simulink model "nonlineardtm"  (R2018b)
settings: configuration reference "Physics" (kept outside this file)
model workspace (MAT data in the model file):
  MCOS : class17 (value not decoded)
undefined symbols (not defined in the file): INIT__initialvalues__Vehicle_InitialPitchAngle, INIT__initialvalues__Vehicle_InitialPitchRate_radps, INIT__initialvalues__Vehicle_InitialVelocity_mps__2, INIT__initialvalues__Vehicle_InitialVelocity_mps__3, INIT__initialvalues__Vehicle_InitialYawAngle, INIT__initialvalues__Vehicle_InitialYawRate_radps, tireFL__INERTIAL__m_Wheel_kg, tireFL__SCALING__LCX, tireFL__SCALING__LCY, tireFL__SCALING__LCZ, tireFL__SCALING__LEX, tireFL__SCALING__LEY, tireFL__SCALING__LFZO, tireFL__SCALING__LGAY, tireFL__SCALING__LGAZ, tireFL__SCALING__LHX, tireFL__SCALING__LHY, tireFL__SCALING__LKX, tireFL__SCALING__LKY, tireFL__SCALING__LMPHI, tireFL__SCALING__LMUV, tireFL__SCALING__LMX, tireFL__SCALING__LMY, tireFL__SCALING__LRES, tireFL__SCALING__LS, tireFL__SCALING__LTR, tireFL__SCALING__LVMX, tireFL__SCALING__LVX, tireFL__SCALING__LVY, tireFL__SCALING__LVYKA, tireFL__SCALING__LXAL, tireFL__SCALING__LYKA, tireFR__INERTIAL__m_Wheel_kg, tireFR__SCALING__LCX, tireFR__SCALING__LCY, tireFR__SCALING__LCZ, tireFR__SCALING__LEX, tireFR__SCALING__LEY, tireFR__SCALING__LFZO, tireFR__SCALING__LGAY, tireFR__SCALING__LGAZ, tireFR__SCALING__LHX, tireFR__SCALING__LHY, tireFR__SCALING__LKX, tireFR__SCALING__LKY, tireFR__SCALING__LMPHI, tireFR__SCALING__LMUV, tireFR__SCALING__LMX, tireFR__SCALING__LMY, tireFR__SCALING__LRES, tireFR__SCALING__LS, tireFR__SCALING__LTR, tireFR__SCALING__LVMX, tireFR__SCALING__LVX, tireFR__SCALING__LVY, tireFR__SCALING__LVYKA, tireFR__SCALING__LXAL, tireFR__SCALING__LYKA, tireRL__INERTIAL__m_Wheel_kg, tireRL__SCALING__LCX ... (+71)
libraries: vehdynlibtire_TUM x4, vehdynlibsuspension x2, vrlib x1, vehdynlibeom_TUM x1
(part 3 of 5)

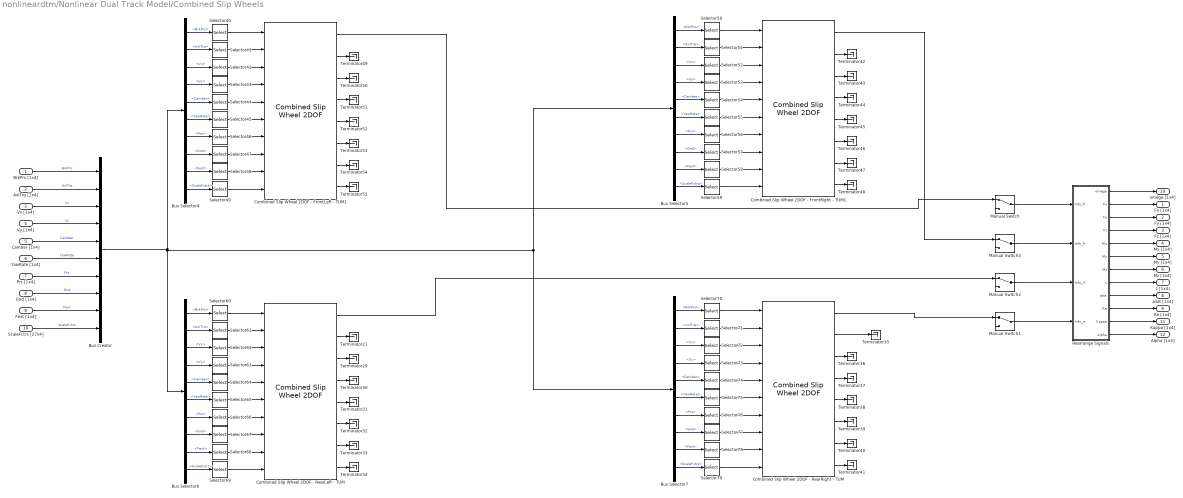
== system nonlineardtm/Nonlinear Dual Track Model/Combined Slip Wheels ==
  BrkPrs [1x4] : Inport
  AxlTrq [1x4] : Inport  Port=2
  Vx [1x4] : Inport  Port=3
  Vy [1x4] : Inport  Port=4
  Camber [1x4] : Inport  Port=5
  YawRate [1x4] : Inport  Port=6
  Prs [1x4] : Inport  Port=7
  Gnd [1x4] : Inport  Port=8
  Fext [1x4] : Inport  Port=9
  ScaleFctrs [27x4] : Inport  Port=10
  Bus Creator : BusCreator  Inputs=10
  Bus Selector{4..7} (4 alike) : BusSelector  OutputSignals=BrkPrs,AxlTrq,Vx,Vy,Camber,YawRate,Prs,Gnd,Fext,ScaleFctrs
  Combined Slip Wheel 2DOF - FrontLeft - TUM1 : vehdynlibtire_TUM/Combined Slip Wheel 2DOF  BrakeType=Disc  mu_static=VEH__Brakes__mue_BrakePadsFrRe_static__1  mu_kinetic=VEH__Brakes__mue_BrakePadsFrRe_kinetic__1  disk_abore=VEH__Brakes__d_BrakeActuatorBoreFrRe_m__1  Rm=VEH__Brakes__r_BrakePadsMeanLeverFrRe_m__1  num_pads=VEH__Brakes__n_BrakePadsNumberFrRe__1  drum_abore=0.0508  drum_a=0.123  drum_c=0.212  drum_r=0.15  drum_theta1=0  drum_theta2=126  brake_p_bpt=[1 11.4736842105263 21.9473684210526 32.4210526315789 42.8947368421053 53.3684210526316 63.8421052631579 74.3157894736842 84.7894736842105 95.2631578947368 105.736842105263 116.210526315789 126.684210526316 137.157894736842 147.631578947368 158.105263157895 168.578947368421 179.052631578947 189.526315789474 200]  brake_n_bpt=[0 52.6315789473684 105.263157894737 157.894736842105 210.526315789474 263.157894736842 315.789473684211 368.421052631579 421.052631578947 473.684210526316 526.315789473684 578.947368421053 631.578947368421 684.210526315789 736.842105263158 789.473684210526 842.105263157895 894.736842105263 947.368421052632 1000]  f_brake_t=[43.4900602404453 42.5056030554862 41.5350898940194 40.5780454442085 39.6340111501808 38.7025443887544 37.7832176914519 36.8756180088306 35.9793460143796 35.0940154454303 34.2192524787115 33.3546951383474 32.4999927342521 31.6548053290159 30.8188032315107 29.991666515561 29.1730845621415 28.362755623661 27.5603864089927 26.765691687993;498.991217495636 487.695866636631 476.560505099801 465.579679307235 454.748127933653 444.060772460445 433.51270824929 423.099196101319 412.81565427025 402.657650900201 392.620896861006 382.701238955775 372.894653477208 363.197240090814 353.605216024701 344.114910546964 334.722759712992 325.425301366216 316.219170376863 307.10109410434;954.492374750826 932.886130217776 911.585920305583 890.581313170261 869.862244717126 849.419000532136 829.242198807128 809.322774193808 789.651962526121 770.221286354971 751.0225412433 732.047782773203 713.289314220164 694.739674852612 676.391628817892 658.238154578366 640.272434863842 622.48784710877 604.877954344734 587.436496520688;1409.99353200602 1378.07639379892 1346.61133551136 1315.58294703329 1284.9763615006 1254.77722860383 1224.97168936497 1195.5463522863 1166.48827078199 1137.78492180974 1109.42418562559 1081.39432659063 1053.68397496312 1026.28210961441 999.178041611083 972.361398609768 945.822110014692 919.550392851325 893.536738312604 867.771898937035;1865.49468926121 1823.26665738007 1781.63675071715 1740.58458089631 1700.09047828407 1660.13545667552 1620.7011799228 1581.76993037878 1543.32457903786 1505.34855726451 1467.82583000789 1430.74087040806 1394.07863570608 1357.82454437621 1321.96445440427 1286.48464264117 1251.37178516554 1216.61293859388 1182.19552228048 1148.10730135338;2320.9958465164 2268.45692096121 2216.66216592293 2165.58621475934 2115.20459506754 2065.49368474721 2016.43067048064 1967.99350847127 1920.16088729373 1872.91219271928 1826.22747439018 1780.08741422549 1734.47329644903 1689.36697913801 1644.75086719747 1600.60788667257 1556.92146031639 1513.67548433643 1470.85430624835 1428.44270376973;2776.49700377159 2713.64718454235 2651.68758112871 2590.58784862237 2530.31871185102 2470.8519128189 2412.16016103848 2354.21708656376 2296.9971955496 2240.47582817405 2184.62911877248 2129.43395804292 2074.86795719199 2020.9094138998 1967.53727999066 1914.73113070398 1862.47113546724 1810.73803007899 1759.51309021622 1708.77810618608;3231.99816102678 3158.8374481235 3086.71299633449 3015.58948248539 2945.43282863449 2876.21014089059 2807.88965159632 2740.44066465625 2673.83350380547 2608.03946362882 2543.03076315477 2478.78050186034 2415.26261793494 2352.4518486616 2290.32369278385 2228.85437473538 2168.02081061809 2107.80057582154 2048.17187418409 1989.11350860242;3687.49931828197 3604.02771170464 3521.73841154027 3440.59111634842 3360.54694541796 3281.56836896228 3203.61914215416 3126.66424274874 3050.66981206134 2975.60309908359 2901.43240753707 2828.12704567777 2755.6572786779 2683.9942834234 2613.11010557704 2542.97761876678 2473.57048576894 2404.8631215641 2336.83065815196 2269.44891101877;4143.00047553716 4049.21797528579 3956.76382674606 3865.59275021144 3775.66106220143 3686.92659703397 3599.34863271199 3512.88782084123 3427.50612031721 3343.16673453836 3259.83405191936 3177.4735894952 3096.05193942085 3015.5367181852 2935.89651837023 2857.10086279818 2779.12016091979 2701.92566730665 2625.48944211983 2549.78431343512;4598.50163279235 4494.40823886693 4391.78924195184 4290.59438407447 4190.77517898491 4092.28482510566 3995.07812326983 3899.11139893372 3804.34242857308 3710.73036999313 3618.23569630166 3526.82013331263 3436.44660016381 3347.079152947 3258.68293116342 3171.22410682959 3084.66983607064 2998.98821304921 2914.1482260877 2830.11971585147;5054.00279004754 4939.59850244808 4826.81465715762 4715.59601793749 4605.88929576838 4497.64305317735 4390.80761382767 4285.3349770262 4181.17873682896 4078.2940054479 3976.63734068395 3876.16667713006 3776.84126090677 3678.62158770879 3581.46934395661 3485.34735086099 ...(+2764 chars)]  tireParamSet=vdynPassCar.mat  plySteer=off  turnslip=off  PRESMAX=tireFL__SIMULATION__PRESMAX  PRESMIN=tireFL__SIMULATION__PRESMIN  FZMAX=tireFL__SIMULATION__FZMAX  FZMIN=tireFL__SIMULATION__FZMIN  VXLOW=tireFL__SIMULATION__VXLOW  KPUMAX=tireFL__SIMULATION__KPUMAX  KPUMIN=tireFL__SIMULATION__KPUMIN  ALPMAX=tireFL__SIMULATION__ALPMAX  ALPMIN=tireFL__SIMULATION__ALPMIN  CAMMAX=tireFL__SIMULATION__CAMMAX  CAMMIN=tireFL__SIMULATION__CAMMIN  LONGVL=tireFL__SIMULATION__LONGVL  omegao=INIT__initialvalues__omega0_Wheels_radps__1  br=tireFL__WHEEL__br_Nmsprad  UNLOADED_RADIUS=tireFL__WHEEL__TYRE_RADIUS_MOD  NOMPRES=tireFL__WHEEL__NORMPRES  FNOMIN=tireFL__WHEEL__FNOMIN  WIDTH=tireFL__DIMENSION__WIDTH  T_RelaxationLong=tireFL__WHEEL__T_RelaxationLong  T_RelaxationLat=tireFL__WHEEL__T_RelaxationLat  T_RelaxationMy=tireFL__WHEEL__T_RelaxationMy  MASS=tireFL__INERTIAL__m_Wheel_kg  IYY=tireFL__INERTIAL__Iyy_Wheel_kgm2  GRAVITY=- VEH__Environment__a_Gravity_mps2  zo=INIT__initialvalues__z0_TireDeflection_m__1  zdoto=INIT__initialvalues__v0z_Wheels_mps__1  BREFF=tireFL__VERTICAL__BREFF  DREFF=tireFL__VERTICAL__DREFF  FREFF=tireFL__VERTICAL__FREFF  Q_RE0=tireFL__VERTICAL__Q_RE0  Q_V1=tireFL__VERTICAL__Q_V1  Q_V2=tireFL__VERTICAL__Q_V2  Q_FZ1=tireFL__VERTICAL__Q_FZ1  Q_FZ2=tireFL__VERTICAL__Q_FZ2  Q_FZ3=tireFL__VERTICAL__Q_FZ3  Q_FCX=tireFL__VERTICAL__Q_FCX  Q_FCY=tireFL__VERTICAL__Q_FCY  Q_FCY2=tireFL__VERTICAL__Q_FCY2  PFZ1=tireFL__VERTICAL__PFZ1  VERTICAL_STIFFNESS=tireFL__VERTICAL__VERTICAL_STIFFNESS  VERTICAL_DAMPING=tireFL__VERTICAL__VERTICAL_DAMPING  LONGITUDINAL_STIFFNESS=tireFL__STRUCTURAL__LONGITUDINAL_STIFFNESS  LATERAL_STIFFNESS=tireFL__STRUCTURAL__LATERAL_STIFFNESS  PCFX1=tireFL__STRUCTURAL__PCFX1  PCFX2=tireFL__STRUCTURAL__PCFX2  PCFX3=tireFL__STRUCTURAL__PCFX3  PCFY1=tireFL__STRUCTURAL__PCFY1  PCFY2=tireFL__STRUCTURAL__PCFY2  PCFY3=tireFL__STRUCTURAL__PCFY3  Q_RA1=tireFL__CONTACTPATCH__Q_RA1  Q_RA2=tireFL__CONTACTPATCH__Q_RA2  Q_RB1=tireFL__CONTACTPATCH__Q_RB1  Q_RB2=tireFL__CONTACTPATCH__Q_RB2  PCX1=tireFL__LONGITUDINAL__PCX1  PDX1=tireFL__LONGITUDINAL__PDX1  PDX2=tireFL__LONGITUDINAL__PDX2  PDX3=tireFL__LONGITUDINAL__PDX3  PEX1=tireFL__LONGITUDINAL__PEX1  PEX2=tireFL__LONGITUDINAL__PEX2  PEX3=tireFL__LONGITUDINAL__PEX3  PEX4=tireFL__LONGITUDINAL__PEX4  PKX1=tireFL__LONGITUDINAL__PKX1  PKX2=tireFL__LONGITUDINAL__PKX2  PKX3=tireFL__LONGITUDINAL__PKX3  PHX1=tireFL__LONGITUDINAL__PHX1  PHX2=tireFL__LONGITUDINAL__PHX2  PVX1=tireFL__LONGITUDINAL__PVX1  PVX2=tireFL__LONGITUDINAL__PVX2  PPX1=tireFL__LONGITUDINAL__PPX1  PPX2=tireFL__LONGITUDINAL__PPX2  PPX3=tireFL__LONGITUDINAL__PPX3  PPX4=tireFL__LONGITUDINAL__PPX4  RBX1=tireFL__LONGITUDINAL__RBX1  RBX2=tireFL__LONGITUDINAL__RBX2  RBX3=tireFL__LONGITUDINAL__RBX3  RCX1=tireFL__LONGITUDINAL__RCX1  REX1=tireFL__LONGITUDINAL__REX1  REX2=tireFL__LONGITUDINAL__REX2  RHX1=tireFL__LONGITUDINAL__RHX1  QSX1=tireFL__OVERTURNING__QSX1  QSX2=tireFL__OVERTURNING__QSX2  QSX3=tireFL__OVERTURNING__QSX3  QSX4=tireFL__OVERTURNING__QSX4  QSX5=tireFL__OVERTURNING__QSX5  QSX6=tireFL__OVERTURNING__QSX6  QSX7=tireFL__OVERTURNING__QSX7  QSX8=tireFL__OVERTURNING__QSX8  QSX9=tireFL__OVERTURNING__QSX9  QSX10=tireFL__OVERTURNING__QSX10  QSX11=tireFL__OVERTURNING__QSX11  QSX12=tireFL__OVERTURNING__QSX12  QSX13=tireFL__OVERTURNING__QSX13  QSX14=tireFL__OVERTURNING__QSX14  PPMX1=tireFL__OVERTURNING__PPMX1  PCY1=tireFL__LATERAL__PCY1  PDY1=tireFL__LATERAL__PDY1  PDY2=tireFL__LATERAL__PDY2  PDY3=tireFL__LATERAL__PDY3  PEY1=tireFL__LATERAL__PEY1  PEY2=tireFL__LATERAL__PEY2  PEY3=tireFL__LATERAL__PEY3  PEY4=tireFL__LATERAL__PEY4  PEY5=tireFL__LATERAL__PEY5  PKY1=tireFL__LATERAL__PKY1  PKY2=tireFL__LATERAL__PKY2  PKY3=tireFL__LATERAL__PKY3  PKY4=tireFL__LATERAL__PKY4  PKY5=tireFL__LATERAL__PKY5  PKY6=tireFL__LATERAL__PKY6  PKY7=tireFL__LATERAL__PKY7  PHY1=tireFL__LATERAL__PHY1  PHY2=tireFL__LATERAL__PHY2  PVY1=tireFL__LATERAL__PVY1  PVY2=tireFL__LATERAL__PVY2  PVY3=tireFL__LATERAL__PVY3  PVY4=tireFL__LATERAL__PVY4  PPY1=tireFL__LATERAL__PPY1  PPY2=tireFL__LATERAL__PPY2  PPY3=tireFL__LATERAL__PPY3  PPY4=tireFL__LATERAL__PPY4  PPY5=tireFL__LATERAL__PPY5  RBY1=tireFL__LATERAL__RBY1  RBY2=tireFL__LATERAL__RBY2  RBY3=tireFL__LATERAL__RBY3  RBY4=tireFL__LATERAL__RBY4  RCY1=tireFL__LATERAL__RCY1  REY1=tireFL__LATERAL__REY1  REY2=tireFL__LATERAL__REY2  RHY1=tireFL__LATERAL__RHY1  RHY2=tireFL__LATERAL__RHY2  RVY1=tireFL__LATERAL__RVY1  RVY2=tireFL__LATERAL__RVY2  RVY3=tireFL__LATERAL__RVY3  RVY4=tireFL__LATERAL__RVY4  RVY5=tireFL__LATERAL__RVY5  RVY6=tireFL__LATERAL__RVY6  QSY1=tireFL__ROLLING__QSY1  QSY2=tireFL__ROLLING__QSY2  QSY3=tireFL__ROLLING__QSY3  QSY4=tireFL__ROLLING__QSY4  QSY5=tireFL__ROLLING__QSY5  QSY6=tireFL__ROLLING__QSY6  QSY7=tireFL__ROLLING__QSY7  QSY8=tireFL__ROLLING__QSY8  QBZ1=tireFL__ALIGNING__QBZ1  QBZ2=tireFL__ALIGNING__QBZ2  QBZ3=tireFL__ALIGNING__QBZ3  QBZ4=tireFL__ALIGNING__QBZ4  QBZ5=tireFL__ALIGNING__QBZ5  QBZ6=tireFL__ALIGNING__QBZ6  QBZ9=tireFL__ALIGNING__QBZ9  QBZ10=tireFL__ALIGNING__QBZ10  QCZ1=tireFL__ALIGNING__QCZ1  QDZ1=tireFL__ALIGNING__QDZ1  QDZ2=tireFL__ALIGNING__QDZ2  QDZ3=tireFL__ALIGNING__QDZ3  QDZ4=tireFL__ALIGNING__QDZ4  QDZ6=tireFL__ALIGNING__QDZ6  QDZ7=tireFL__ALIGNING__QDZ7  QDZ8=tireFL__ALIGNING__QDZ8  QDZ9=tireFL__ALIGNING__QDZ9  QDZ10=tireFL__ALIGNING__QDZ10  QDZ11=tireFL__ALIGNING__QDZ11  QEZ1=tireFL__ALIGNING__QEZ1  QEZ2=tireFL__ALIGNING__QEZ2  QEZ3=tireFL__ALIGNING__QEZ3  QEZ4=tireFL__ALIGNING__QEZ4  QEZ5=tireFL__ALIGNING__QEZ5  QHZ1=tireFL__ALIGNING__QHZ1  QHZ2=tireFL__ALIGNING__QHZ2  QHZ3=tireFL__ALIGNING__QHZ3  QHZ4=tireFL__ALIGNING__QHZ4  PPZ1=tireFL__ALIGNING__PPZ1  PPZ2=tireFL__ALIGNING__PPZ2  SSZ1=tireFL__ALIGNING__SSZ1  SSZ2=tireFL__ALIGNING__SSZ2  SSZ3=tireFL__ALIGNING__SSZ3  SSZ4=tireFL__ALIGNING__SSZ4  PDXP1=tireFL__TURNSLIP__PDXP1  PDXP2=tireFL__TURNSLIP__PDXP2  PDXP3=tireFL__TURNSLIP__PDXP3  PKYP1=tireFL__TURNSLIP__PKYP1  PDYP1=tireFL__TURNSLIP__PDYP1  PDYP2=tireFL__TURNSLIP__PDYP2  PDYP3=tireFL__TURNSLIP__PDYP3  PDYP4=tireFL__TURNSLIP__PDYP4  PHYP1=tireFL__TURNSLIP__PHYP1  PHYP2=tireFL__TURNSLIP__PHYP2  PHYP3=tireFL__TURNSLIP__PHYP3  PHYP4=tireFL__TURNSLIP__PHYP4  PECP1=tireFL__TURNSLIP__PECP1  PECP2=tireFL__TURNSLIP__PECP2  QDTP1=tireFL__TURNSLIP__QDTP1  QCRP1=tireFL__TURNSLIP__QCRP1  QCRP2=tireFL__TURNSLIP__QCRP2  QBRP1=tireFL__TURNSLIP__QBRP1  QDRP1=tireFL__TURNSLIP__QDRP1  QDRP2=tireFL__TURNSLIP__QDRP2  aMode=2
  Combined Slip Wheel 2DOF - FrontRight - TUM1 : vehdynlibtire_TUM/Combined Slip Wheel 2DOF  BrakeType=Disc  mu_static=VEH__Brakes__mue_BrakePadsFrRe_static__1  mu_kinetic=VEH__Brakes__mue_BrakePadsFrRe_kinetic__1  disk_abore=VEH__Brakes__d_BrakeActuatorBoreFrRe_m__1  Rm=VEH__Brakes__r_BrakePadsMeanLeverFrRe_m__1  num_pads=VEH__Brakes__n_BrakePadsNumberFrRe__1  drum_abore=0.0508  drum_a=0.123  drum_c=0.212  drum_r=0.15  drum_theta1=0  drum_theta2=126  brake_p_bpt=[1 11.4736842105263 21.9473684210526 32.4210526315789 42.8947368421053 53.3684210526316 63.8421052631579 74.3157894736842 84.7894736842105 95.2631578947368 105.736842105263 116.210526315789 126.684210526316 137.157894736842 147.631578947368 158.105263157895 168.578947368421 179.052631578947 189.526315789474 200]  brake_n_bpt=[0 52.6315789473684 105.263157894737 157.894736842105 210.526315789474 263.157894736842 315.789473684211 368.421052631579 421.052631578947 473.684210526316 526.315789473684 578.947368421053 631.578947368421 684.210526315789 736.842105263158 789.473684210526 842.105263157895 894.736842105263 947.368421052632 1000]  f_brake_t=[43.4900602404453 42.5056030554862 41.5350898940194 40.5780454442085 39.6340111501808 38.7025443887544 37.7832176914519 36.8756180088306 35.9793460143796 35.0940154454303 34.2192524787115 33.3546951383474 32.4999927342521 31.6548053290159 30.8188032315107 29.991666515561 29.1730845621415 28.362755623661 27.5603864089927 26.765691687993;498.991217495636 487.695866636631 476.560505099801 465.579679307235 454.748127933653 444.060772460445 433.51270824929 423.099196101319 412.81565427025 402.657650900201 392.620896861006 382.701238955775 372.894653477208 363.197240090814 353.605216024701 344.114910546964 334.722759712992 325.425301366216 316.219170376863 307.10109410434;954.492374750826 932.886130217776 911.585920305583 890.581313170261 869.862244717126 849.419000532136 829.242198807128 809.322774193808 789.651962526121 770.221286354971 751.0225412433 732.047782773203 713.289314220164 694.739674852612 676.391628817892 658.238154578366 640.272434863842 622.48784710877 604.877954344734 587.436496520688;1409.99353200602 1378.07639379892 1346.61133551136 1315.58294703329 1284.9763615006 1254.77722860383 1224.97168936497 1195.5463522863 1166.48827078199 1137.78492180974 1109.42418562559 1081.39432659063 1053.68397496312 1026.28210961441 999.178041611083 972.361398609768 945.822110014692 919.550392851325 893.536738312604 867.771898937035;1865.49468926121 1823.26665738007 1781.63675071715 1740.58458089631 1700.09047828407 1660.13545667552 1620.7011799228 1581.76993037878 1543.32457903786 1505.34855726451 1467.82583000789 1430.74087040806 1394.07863570608 1357.82454437621 1321.96445440427 1286.48464264117 1251.37178516554 1216.61293859388 1182.19552228048 1148.10730135338;2320.9958465164 2268.45692096121 2216.66216592293 2165.58621475934 2115.20459506754 2065.49368474721 2016.43067048064 1967.99350847127 1920.16088729373 1872.91219271928 1826.22747439018 1780.08741422549 1734.47329644903 1689.36697913801 1644.75086719747 1600.60788667257 1556.92146031639 1513.67548433643 1470.85430624835 1428.44270376973;2776.49700377159 2713.64718454235 2651.68758112871 2590.58784862237 2530.31871185102 2470.8519128189 2412.16016103848 2354.21708656376 2296.9971955496 2240.47582817405 2184.62911877248 2129.43395804292 2074.86795719199 2020.9094138998 1967.53727999066 1914.73113070398 1862.47113546724 1810.73803007899 1759.51309021622 1708.77810618608;3231.99816102678 3158.8374481235 3086.71299633449 3015.58948248539 2945.43282863449 2876.21014089059 2807.88965159632 2740.44066465625 2673.83350380547 2608.03946362882 2543.03076315477 2478.78050186034 2415.26261793494 2352.4518486616 2290.32369278385 2228.85437473538 2168.02081061809 2107.80057582154 2048.17187418409 1989.11350860242;3687.49931828197 3604.02771170464 3521.73841154027 3440.59111634842 3360.54694541796 3281.56836896228 3203.61914215416 3126.66424274874 3050.66981206134 2975.60309908359 2901.43240753707 2828.12704567777 2755.6572786779 2683.9942834234 2613.11010557704 2542.97761876678 2473.57048576894 2404.8631215641 2336.83065815196 2269.44891101877;4143.00047553716 4049.21797528579 3956.76382674606 3865.59275021144 3775.66106220143 3686.92659703397 3599.34863271199 3512.88782084123 3427.50612031721 3343.16673453836 3259.83405191936 3177.4735894952 3096.05193942085 3015.5367181852 2935.89651837023 2857.10086279818 2779.12016091979 2701.92566730665 2625.48944211983 2549.78431343512;4598.50163279235 4494.40823886693 4391.78924195184 4290.59438407447 4190.77517898491 4092.28482510566 3995.07812326983 3899.11139893372 3804.34242857308 3710.73036999313 3618.23569630166 3526.82013331263 3436.44660016381 3347.079152947 3258.68293116342 3171.22410682959 3084.66983607064 2998.98821304921 2914.1482260877 2830.11971585147;5054.00279004754 4939.59850244808 4826.81465715762 4715.59601793749 4605.88929576838 4497.64305317735 4390.80761382767 4285.3349770262 4181.17873682896 4078.2940054479 3976.63734068395 3876.16667713006 3776.84126090677 3678.62158770879 3581.46934395661 3485.34735086099 ...(+2764 chars)]  tireParamSet=vdynPassCar.mat  plySteer=off  turnslip=off  PRESMAX=tireFR__SIMULATION__PRESMAX  PRESMIN=tireFR__SIMULATION__PRESMIN  FZMAX=tireFR__SIMULATION__FZMAX  FZMIN=tireFR__SIMULATION__FZMIN  VXLOW=tireFR__SIMULATION__VXLOW  KPUMAX=tireFR__SIMULATION__KPUMAX  KPUMIN=tireFR__SIMULATION__KPUMIN  ALPMAX=tireFR__SIMULATION__ALPMAX  ALPMIN=tireFR__SIMULATION__ALPMIN  CAMMAX=tireFR__SIMULATION__CAMMAX  CAMMIN=tireFR__SIMULATION__CAMMIN  LONGVL=tireFR__SIMULATION__LONGVL  omegao=INIT__initialvalues__omega0_Wheels_radps__2  br=tireFR__WHEEL__br_Nmsprad  UNLOADED_RADIUS=tireFR__WHEEL__TYRE_RADIUS_MOD  NOMPRES=tireFR__WHEEL__NORMPRES  FNOMIN=tireFR__WHEEL__FNOMIN  WIDTH=tireFR__DIMENSION__WIDTH  T_RelaxationLong=tireFR__WHEEL__T_RelaxationLong  T_RelaxationLat=tireFR__WHEEL__T_RelaxationLat  T_RelaxationMy=tireFR__WHEEL__T_RelaxationMy  MASS=tireFR__INERTIAL__m_Wheel_kg  IYY=tireFR__INERTIAL__Iyy_Wheel_kgm2  GRAVITY=- VEH__Environment__a_Gravity_mps2  zo=INIT__initialvalues__z0_TireDeflection_m__2  zdoto=INIT__initialvalues__v0z_Wheels_mps__2  BREFF=tireFR__VERTICAL__BREFF  DREFF=tireFR__VERTICAL__DREFF  FREFF=tireFR__VERTICAL__FREFF  Q_RE0=tireFR__VERTICAL__Q_RE0  Q_V1=tireFR__VERTICAL__Q_V1  Q_V2=tireFR__VERTICAL__Q_V2  Q_FZ1=tireFR__VERTICAL__Q_FZ1  Q_FZ2=tireFR__VERTICAL__Q_FZ2  Q_FZ3=tireFR__VERTICAL__Q_FZ3  Q_FCX=tireFR__VERTICAL__Q_FCX  Q_FCY=tireFR__VERTICAL__Q_FCY  Q_FCY2=tireFR__VERTICAL__Q_FCY2  PFZ1=tireFR__VERTICAL__PFZ1  VERTICAL_STIFFNESS=tireFR__VERTICAL__VERTICAL_STIFFNESS  VERTICAL_DAMPING=tireFR__VERTICAL__VERTICAL_DAMPING  LONGITUDINAL_STIFFNESS=tireFR__STRUCTURAL__LONGITUDINAL_STIFFNESS  LATERAL_STIFFNESS=tireFR__STRUCTURAL__LATERAL_STIFFNESS  PCFX1=tireFR__STRUCTURAL__PCFX1  PCFX2=tireFR__STRUCTURAL__PCFX2  PCFX3=tireFR__STRUCTURAL__PCFX3  PCFY1=tireFR__STRUCTURAL__PCFY1  PCFY2=tireFR__STRUCTURAL__PCFY2  PCFY3=tireFR__STRUCTURAL__PCFY3  Q_RA1=tireFR__CONTACTPATCH__Q_RA1  Q_RA2=tireFR__CONTACTPATCH__Q_RA2  Q_RB1=tireFR__CONTACTPATCH__Q_RB1  Q_RB2=tireFR__CONTACTPATCH__Q_RB2  PCX1=tireFR__LONGITUDINAL__PCX1  PDX1=tireFR__LONGITUDINAL__PDX1  PDX2=tireFR__LONGITUDINAL__PDX2  PDX3=tireFR__LONGITUDINAL__PDX3  PEX1=tireFR__LONGITUDINAL__PEX1  PEX2=tireFR__LONGITUDINAL__PEX2  PEX3=tireFR__LONGITUDINAL__PEX3  PEX4=tireFR__LONGITUDINAL__PEX4  PKX1=tireFR__LONGITUDINAL__PKX1  PKX2=tireFR__LONGITUDINAL__PKX2  PKX3=tireFR__LONGITUDINAL__PKX3  PHX1=tireFR__LONGITUDINAL__PHX1  PHX2=tireFR__LONGITUDINAL__PHX2  PVX1=tireFR__LONGITUDINAL__PVX1  PVX2=tireFR__LONGITUDINAL__PVX2  PPX1=tireFR__LONGITUDINAL__PPX1  PPX2=tireFR__LONGITUDINAL__PPX2  PPX3=tireFR__LONGITUDINAL__PPX3  PPX4=tireFR__LONGITUDINAL__PPX4  RBX1=tireFR__LONGITUDINAL__RBX1  RBX2=tireFR__LONGITUDINAL__RBX2  RBX3=tireFR__LONGITUDINAL__RBX3  RCX1=tireFR__LONGITUDINAL__RCX1  REX1=tireFR__LONGITUDINAL__REX1  REX2=tireFR__LONGITUDINAL__REX2  RHX1=tireFR__LONGITUDINAL__RHX1  QSX1=tireFR__OVERTURNING__QSX1  QSX2=tireFR__OVERTURNING__QSX2  QSX3=tireFR__OVERTURNING__QSX3  QSX4=tireFR__OVERTURNING__QSX4  QSX5=tireFR__OVERTURNING__QSX5  QSX6=tireFR__OVERTURNING__QSX6  QSX7=tireFR__OVERTURNING__QSX7  QSX8=tireFR__OVERTURNING__QSX8  QSX9=tireFR__OVERTURNING__QSX9  QSX10=tireFR__OVERTURNING__QSX10  QSX11=tireFR__OVERTURNING__QSX11  QSX12=tireFR__OVERTURNING__QSX12  QSX13=tireFR__OVERTURNING__QSX13  QSX14=tireFR__OVERTURNING__QSX14  PPMX1=tireFR__OVERTURNING__PPMX1  PCY1=tireFR__LATERAL__PCY1  PDY1=tireFR__LATERAL__PDY1  PDY2=tireFR__LATERAL__PDY2  PDY3=tireFR__LATERAL__PDY3  PEY1=tireFR__LATERAL__PEY1  PEY2=tireFR__LATERAL__PEY2  PEY3=tireFR__LATERAL__PEY3  PEY4=tireFR__LATERAL__PEY4  PEY5=tireFR__LATERAL__PEY5  PKY1=tireFR__LATERAL__PKY1  PKY2=tireFR__LATERAL__PKY2  PKY3=tireFR__LATERAL__PKY3  PKY4=tireFR__LATERAL__PKY4  PKY5=tireFR__LATERAL__PKY5  PKY6=tireFR__LATERAL__PKY6  PKY7=tireFR__LATERAL__PKY7  PHY1=tireFR__LATERAL__PHY1  PHY2=tireFR__LATERAL__PHY2  PVY1=tireFR__LATERAL__PVY1  PVY2=tireFR__LATERAL__PVY2  PVY3=tireFR__LATERAL__PVY3  PVY4=tireFR__LATERAL__PVY4  PPY1=tireFR__LATERAL__PPY1  PPY2=tireFR__LATERAL__PPY2  PPY3=tireFR__LATERAL__PPY3  PPY4=tireFR__LATERAL__PPY4  PPY5=tireFR__LATERAL__PPY5  RBY1=tireFR__LATERAL__RBY1  RBY2=tireFR__LATERAL__RBY2  RBY3=tireFR__LATERAL__RBY3  RBY4=tireFR__LATERAL__RBY4  RCY1=tireFR__LATERAL__RCY1  REY1=tireFR__LATERAL__REY1  REY2=tireFR__LATERAL__REY2  RHY1=tireFR__LATERAL__RHY1  RHY2=tireFR__LATERAL__RHY2  RVY1=tireFR__LATERAL__RVY1  RVY2=tireFR__LATERAL__RVY2  RVY3=tireFR__LATERAL__RVY3  RVY4=tireFR__LATERAL__RVY4  RVY5=tireFR__LATERAL__RVY5  RVY6=tireFR__LATERAL__RVY6  QSY1=tireFR__ROLLING__QSY1  QSY2=tireFR__ROLLING__QSY2  QSY3=tireFR__ROLLING__QSY3  QSY4=tireFR__ROLLING__QSY4  QSY5=tireFR__ROLLING__QSY5  QSY6=tireFR__ROLLING__QSY6  QSY7=tireFR__ROLLING__QSY7  QSY8=tireFR__ROLLING__QSY8  QBZ1=tireFR__ALIGNING__QBZ1  QBZ2=tireFR__ALIGNING__QBZ2  QBZ3=tireFR__ALIGNING__QBZ3  QBZ4=tireFR__ALIGNING__QBZ4  QBZ5=tireFR__ALIGNING__QBZ5  QBZ6=tireFR__ALIGNING__QBZ6  QBZ9=tireFR__ALIGNING__QBZ9  QBZ10=tireFR__ALIGNING__QBZ10  QCZ1=tireFR__ALIGNING__QCZ1  QDZ1=tireFR__ALIGNING__QDZ1  QDZ2=tireFR__ALIGNING__QDZ2  QDZ3=tireFR__ALIGNING__QDZ3  QDZ4=tireFR__ALIGNING__QDZ4  QDZ6=tireFR__ALIGNING__QDZ6  QDZ7=tireFR__ALIGNING__QDZ7  QDZ8=tireFR__ALIGNING__QDZ8  QDZ9=tireFR__ALIGNING__QDZ9  QDZ10=tireFR__ALIGNING__QDZ10  QDZ11=tireFR__ALIGNING__QDZ11  QEZ1=tireFR__ALIGNING__QEZ1  QEZ2=tireFR__ALIGNING__QEZ2  QEZ3=tireFR__ALIGNING__QEZ3  QEZ4=tireFR__ALIGNING__QEZ4  QEZ5=tireFR__ALIGNING__QEZ5  QHZ1=tireFR__ALIGNING__QHZ1  QHZ2=tireFR__ALIGNING__QHZ2  QHZ3=tireFR__ALIGNING__QHZ3  QHZ4=tireFR__ALIGNING__QHZ4  PPZ1=tireFR__ALIGNING__PPZ1  PPZ2=tireFR__ALIGNING__PPZ2  SSZ1=tireFR__ALIGNING__SSZ1  SSZ2=tireFR__ALIGNING__SSZ2  SSZ3=tireFR__ALIGNING__SSZ3  SSZ4=tireFR__ALIGNING__SSZ4  PDXP1=tireFR__TURNSLIP__PDXP1  PDXP2=tireFR__TURNSLIP__PDXP2  PDXP3=tireFR__TURNSLIP__PDXP3  PKYP1=tireFR__TURNSLIP__PKYP1  PDYP1=tireFR__TURNSLIP__PDYP1  PDYP2=tireFR__TURNSLIP__PDYP2  PDYP3=tireFR__TURNSLIP__PDYP3  PDYP4=tireFR__TURNSLIP__PDYP4  PHYP1=tireFR__TURNSLIP__PHYP1  PHYP2=tireFR__TURNSLIP__PHYP2  PHYP3=tireFR__TURNSLIP__PHYP3  PHYP4=tireFR__TURNSLIP__PHYP4  PECP1=tireFR__TURNSLIP__PECP1  PECP2=tireFR__TURNSLIP__PECP2  QDTP1=tireFR__TURNSLIP__QDTP1  QCRP1=tireFR__TURNSLIP__QCRP1  QCRP2=tireFR__TURNSLIP__QCRP2  QBRP1=tireFR__TURNSLIP__QBRP1  QDRP1=tireFR__TURNSLIP__QDRP1  QDRP2=tireFR__TURNSLIP__QDRP2  aMode=2
  Combined Slip Wheel 2DOF - RearLeft - TUM : vehdynlibtire_TUM/Combined Slip Wheel 2DOF  BrakeType=Disc  mu_static=VEH__Brakes__mue_BrakePadsFrRe_static__2  mu_kinetic=VEH__Brakes__mue_BrakePadsFrRe_kinetic__2  disk_abore=VEH__Brakes__d_BrakeActuatorBoreFrRe_m__2  Rm=VEH__Brakes__r_BrakePadsMeanLeverFrRe_m__2  num_pads=VEH__Brakes__n_BrakePadsNumberFrRe__2  drum_abore=0.0508  drum_a=0.123  drum_c=0.212  drum_r=0.15  drum_theta1=0  drum_theta2=126  brake_p_bpt=[1 11.4736842105263 21.9473684210526 32.4210526315789 42.8947368421053 53.3684210526316 63.8421052631579 74.3157894736842 84.7894736842105 95.2631578947368 105.736842105263 116.210526315789 126.684210526316 137.157894736842 147.631578947368 158.105263157895 168.578947368421 179.052631578947 189.526315789474 200]  brake_n_bpt=[0 52.6315789473684 105.263157894737 157.894736842105 210.526315789474 263.157894736842 315.789473684211 368.421052631579 421.052631578947 473.684210526316 526.315789473684 578.947368421053 631.578947368421 684.210526315789 736.842105263158 789.473684210526 842.105263157895 894.736842105263 947.368421052632 1000]  f_brake_t=[43.4900602404453 42.5056030554862 41.5350898940194 40.5780454442085 39.6340111501808 38.7025443887544 37.7832176914519 36.8756180088306 35.9793460143796 35.0940154454303 34.2192524787115 33.3546951383474 32.4999927342521 31.6548053290159 30.8188032315107 29.991666515561 29.1730845621415 28.362755623661 27.5603864089927 26.765691687993;498.991217495636 487.695866636631 476.560505099801 465.579679307235 454.748127933653 444.060772460445 433.51270824929 423.099196101319 412.81565427025 402.657650900201 392.620896861006 382.701238955775 372.894653477208 363.197240090814 353.605216024701 344.114910546964 334.722759712992 325.425301366216 316.219170376863 307.10109410434;954.492374750826 932.886130217776 911.585920305583 890.581313170261 869.862244717126 849.419000532136 829.242198807128 809.322774193808 789.651962526121 770.221286354971 751.0225412433 732.047782773203 713.289314220164 694.739674852612 676.391628817892 658.238154578366 640.272434863842 622.48784710877 604.877954344734 587.436496520688;1409.99353200602 1378.07639379892 1346.61133551136 1315.58294703329 1284.9763615006 1254.77722860383 1224.97168936497 1195.5463522863 1166.48827078199 1137.78492180974 1109.42418562559 1081.39432659063 1053.68397496312 1026.28210961441 999.178041611083 972.361398609768 945.822110014692 919.550392851325 893.536738312604 867.771898937035;1865.49468926121 1823.26665738007 1781.63675071715 1740.58458089631 1700.09047828407 1660.13545667552 1620.7011799228 1581.76993037878 1543.32457903786 1505.34855726451 1467.82583000789 1430.74087040806 1394.07863570608 1357.82454437621 1321.96445440427 1286.48464264117 1251.37178516554 1216.61293859388 1182.19552228048 1148.10730135338;2320.9958465164 2268.45692096121 2216.66216592293 2165.58621475934 2115.20459506754 2065.49368474721 2016.43067048064 1967.99350847127 1920.16088729373 1872.91219271928 1826.22747439018 1780.08741422549 1734.47329644903 1689.36697913801 1644.75086719747 1600.60788667257 1556.92146031639 1513.67548433643 1470.85430624835 1428.44270376973;2776.49700377159 2713.64718454235 2651.68758112871 2590.58784862237 2530.31871185102 2470.8519128189 2412.16016103848 2354.21708656376 2296.9971955496 2240.47582817405 2184.62911877248 2129.43395804292 2074.86795719199 2020.9094138998 1967.53727999066 1914.73113070398 1862.47113546724 1810.73803007899 1759.51309021622 1708.77810618608;3231.99816102678 3158.8374481235 3086.71299633449 3015.58948248539 2945.43282863449 2876.21014089059 2807.88965159632 2740.44066465625 2673.83350380547 2608.03946362882 2543.03076315477 2478.78050186034 2415.26261793494 2352.4518486616 2290.32369278385 2228.85437473538 2168.02081061809 2107.80057582154 2048.17187418409 1989.11350860242;3687.49931828197 3604.02771170464 3521.73841154027 3440.59111634842 3360.54694541796 3281.56836896228 3203.61914215416 3126.66424274874 3050.66981206134 2975.60309908359 2901.43240753707 2828.12704567777 2755.6572786779 2683.9942834234 2613.11010557704 2542.97761876678 2473.57048576894 2404.8631215641 2336.83065815196 2269.44891101877;4143.00047553716 4049.21797528579 3956.76382674606 3865.59275021144 3775.66106220143 3686.92659703397 3599.34863271199 3512.88782084123 3427.50612031721 3343.16673453836 3259.83405191936 3177.4735894952 3096.05193942085 3015.5367181852 2935.89651837023 2857.10086279818 2779.12016091979 2701.92566730665 2625.48944211983 2549.78431343512;4598.50163279235 4494.40823886693 4391.78924195184 4290.59438407447 4190.77517898491 4092.28482510566 3995.07812326983 3899.11139893372 3804.34242857308 3710.73036999313 3618.23569630166 3526.82013331263 3436.44660016381 3347.079152947 3258.68293116342 3171.22410682959 3084.66983607064 2998.98821304921 2914.1482260877 2830.11971585147;5054.00279004754 4939.59850244808 4826.81465715762 4715.59601793749 4605.88929576838 4497.64305317735 4390.80761382767 4285.3349770262 4181.17873682896 4078.2940054479 3976.63734068395 3876.16667713006 3776.84126090677 3678.62158770879 3581.46934395661 3485.34735086099 ...(+2764 chars)]  tireParamSet=vdynPassCar.mat  plySteer=off  turnslip=off  PRESMAX=tireRL__SIMULATION__PRESMAX  PRESMIN=tireRL__SIMULATION__PRESMIN  FZMAX=tireRL__SIMULATION__FZMAX  FZMIN=tireRL__SIMULATION__FZMIN  VXLOW=tireRL__SIMULATION__VXLOW  KPUMAX=tireRL__SIMULATION__KPUMAX  KPUMIN=tireRL__SIMULATION__KPUMIN  ALPMAX=tireRL__SIMULATION__ALPMAX  ALPMIN=tireRL__SIMULATION__ALPMIN  CAMMAX=tireRL__SIMULATION__CAMMAX  CAMMIN=tireRL__SIMULATION__CAMMIN  LONGVL=tireRL__SIMULATION__LONGVL  omegao=INIT__initialvalues__omega0_Wheels_radps__3  br=tireRL__WHEEL__br_Nmsprad  UNLOADED_RADIUS=tireRL__WHEEL__TYRE_RADIUS_MOD  NOMPRES=tireRL__WHEEL__NORMPRES  FNOMIN=tireRL__WHEEL__FNOMIN  WIDTH=tireRL__DIMENSION__WIDTH  T_RelaxationLong=tireRL__WHEEL__T_RelaxationLong  T_RelaxationLat=tireRL__WHEEL__T_RelaxationLat  T_RelaxationMy=tireRL__WHEEL__T_RelaxationMy  MASS=tireRL__INERTIAL__m_Wheel_kg  IYY=tireRL__INERTIAL__Iyy_Wheel_kgm2  GRAVITY=- VEH__Environment__a_Gravity_mps2  zo=INIT__initialvalues__z0_TireDeflection_m__3  zdoto=INIT__initialvalues__v0z_Wheels_mps__3  BREFF=tireRL__VERTICAL__BREFF  DREFF=tireRL__VERTICAL__DREFF  FREFF=tireRL__VERTICAL__FREFF  Q_RE0=tireRL__VERTICAL__Q_RE0  Q_V1=tireRL__VERTICAL__Q_V1  Q_V2=tireRL__VERTICAL__Q_V2  Q_FZ1=tireRL__VERTICAL__Q_FZ1  Q_FZ2=tireRL__VERTICAL__Q_FZ2  Q_FZ3=tireRL__VERTICAL__Q_FZ3  Q_FCX=tireRL__VERTICAL__Q_FCX  Q_FCY=tireRL__VERTICAL__Q_FCY  Q_FCY2=tireRL__VERTICAL__Q_FCY2  PFZ1=tireRL__VERTICAL__PFZ1  VERTICAL_STIFFNESS=tireRL__VERTICAL__VERTICAL_STIFFNESS  VERTICAL_DAMPING=tireRL__VERTICAL__VERTICAL_DAMPING  LONGITUDINAL_STIFFNESS=tireRL__STRUCTURAL__LONGITUDINAL_STIFFNESS  LATERAL_STIFFNESS=tireRL__STRUCTURAL__LATERAL_STIFFNESS  PCFX1=tireRL__STRUCTURAL__PCFX1  PCFX2=tireRL__STRUCTURAL__PCFX2  PCFX3=tireRL__STRUCTURAL__PCFX3  PCFY1=tireRL__STRUCTURAL__PCFY1  PCFY2=tireRL__STRUCTURAL__PCFY2  PCFY3=tireRL__STRUCTURAL__PCFY3  Q_RA1=tireRL__CONTACTPATCH__Q_RA1  Q_RA2=tireRL__CONTACTPATCH__Q_RA2  Q_RB1=tireRL__CONTACTPATCH__Q_RB1  Q_RB2=tireRL__CONTACTPATCH__Q_RB2  PCX1=tireRL__LONGITUDINAL__PCX1  PDX1=tireRL__LONGITUDINAL__PDX1  PDX2=tireRL__LONGITUDINAL__PDX2  PDX3=tireRL__LONGITUDINAL__PDX3  PEX1=tireRL__LONGITUDINAL__PEX1  PEX2=tireRL__LONGITUDINAL__PEX2  PEX3=tireRL__LONGITUDINAL__PEX3  PEX4=tireRL__LONGITUDINAL__PEX4  PKX1=tireRL__LONGITUDINAL__PKX1  PKX2=tireRL__LONGITUDINAL__PKX2  PKX3=tireRL__LONGITUDINAL__PKX3  PHX1=tireRL__LONGITUDINAL__PHX1  PHX2=tireRL__LONGITUDINAL__PHX2  PVX1=tireRL__LONGITUDINAL__PVX1  PVX2=tireRL__LONGITUDINAL__PVX2  PPX1=tireRL__LONGITUDINAL__PPX1  PPX2=tireRL__LONGITUDINAL__PPX2  PPX3=tireRL__LONGITUDINAL__PPX3  PPX4=tireRL__LONGITUDINAL__PPX4  RBX1=tireRL__LONGITUDINAL__RBX1  RBX2=tireRL__LONGITUDINAL__RBX2  RBX3=tireRL__LONGITUDINAL__RBX3  RCX1=tireRL__LONGITUDINAL__RCX1  REX1=tireRL__LONGITUDINAL__REX1  REX2=tireRL__LONGITUDINAL__REX2  RHX1=tireRL__LONGITUDINAL__RHX1  QSX1=tireRL__OVERTURNING__QSX1  QSX2=tireRL__OVERTURNING__QSX2  QSX3=tireRL__OVERTURNING__QSX3  QSX4=tireRL__OVERTURNING__QSX4  QSX5=tireRL__OVERTURNING__QSX5  QSX6=tireRL__OVERTURNING__QSX6  QSX7=tireRL__OVERTURNING__QSX7  QSX8=tireRL__OVERTURNING__QSX8  QSX9=tireRL__OVERTURNING__QSX9  QSX10=tireRL__OVERTURNING__QSX10  QSX11=tireRL__OVERTURNING__QSX11  QSX12=tireRL__OVERTURNING__QSX12  QSX13=tireRL__OVERTURNING__QSX13  QSX14=tireRL__OVERTURNING__QSX14  PPMX1=tireRL__OVERTURNING__PPMX1  PCY1=tireRL__LATERAL__PCY1  PDY1=tireRL__LATERAL__PDY1  PDY2=tireRL__LATERAL__PDY2  PDY3=tireRL__LATERAL__PDY3  PEY1=tireRL__LATERAL__PEY1  PEY2=tireRL__LATERAL__PEY2  PEY3=tireRL__LATERAL__PEY3  PEY4=tireRL__LATERAL__PEY4  PEY5=tireRL__LATERAL__PEY5  PKY1=tireRL__LATERAL__PKY1  PKY2=tireRL__LATERAL__PKY2  PKY3=tireRL__LATERAL__PKY3  PKY4=tireRL__LATERAL__PKY4  PKY5=tireRL__LATERAL__PKY5  PKY6=tireRL__LATERAL__PKY6  PKY7=tireRL__LATERAL__PKY7  PHY1=tireRL__LATERAL__PHY1  PHY2=tireRL__LATERAL__PHY2  PVY1=tireRL__LATERAL__PVY1  PVY2=tireRL__LATERAL__PVY2  PVY3=tireRL__LATERAL__PVY3  PVY4=tireRL__LATERAL__PVY4  PPY1=tireRL__LATERAL__PPY1  PPY2=tireRL__LATERAL__PPY2  PPY3=tireRL__LATERAL__PPY3  PPY4=tireRL__LATERAL__PPY4  PPY5=tireRL__LATERAL__PPY5  RBY1=tireRL__LATERAL__RBY1  RBY2=tireRL__LATERAL__RBY2  RBY3=tireRL__LATERAL__RBY3  RBY4=tireRL__LATERAL__RBY4  RCY1=tireRL__LATERAL__RCY1  REY1=tireRL__LATERAL__REY1  REY2=tireRL__LATERAL__REY2  RHY1=tireRL__LATERAL__RHY1  RHY2=tireRL__LATERAL__RHY2  RVY1=tireRL__LATERAL__RVY1  RVY2=tireRL__LATERAL__RVY2  RVY3=tireRL__LATERAL__RVY3  RVY4=tireRL__LATERAL__RVY4  RVY5=tireRL__LATERAL__RVY5  RVY6=tireRL__LATERAL__RVY6  QSY1=tireRL__ROLLING__QSY1  QSY2=tireRL__ROLLING__QSY2  QSY3=tireRL__ROLLING__QSY3  QSY4=tireRL__ROLLING__QSY4  QSY5=tireRL__ROLLING__QSY5  QSY6=tireRL__ROLLING__QSY6  QSY7=tireRL__ROLLING__QSY7  QSY8=tireRL__ROLLING__QSY8  QBZ1=tireRL__ALIGNING__QBZ1  QBZ2=tireRL__ALIGNING__QBZ2  QBZ3=tireRL__ALIGNING__QBZ3  QBZ4=tireRL__ALIGNING__QBZ4  QBZ5=tireRL__ALIGNING__QBZ5  QBZ6=tireRL__ALIGNING__QBZ6  QBZ9=tireRL__ALIGNING__QBZ9  QBZ10=tireRL__ALIGNING__QBZ10  QCZ1=tireRL__ALIGNING__QCZ1  QDZ1=tireRL__ALIGNING__QDZ1  QDZ2=tireRL__ALIGNING__QDZ2  QDZ3=tireRL__ALIGNING__QDZ3  QDZ4=tireRL__ALIGNING__QDZ4  QDZ6=tireRL__ALIGNING__QDZ6  QDZ7=tireRL__ALIGNING__QDZ7  QDZ8=tireRL__ALIGNING__QDZ8  QDZ9=tireRL__ALIGNING__QDZ9  QDZ10=tireRL__ALIGNING__QDZ10  QDZ11=tireRL__ALIGNING__QDZ11  QEZ1=tireRL__ALIGNING__QEZ1  QEZ2=tireRL__ALIGNING__QEZ2  QEZ3=tireRL__ALIGNING__QEZ3  QEZ4=tireRL__ALIGNING__QEZ4  QEZ5=tireRL__ALIGNING__QEZ5  QHZ1=tireRL__ALIGNING__QHZ1  QHZ2=tireRL__ALIGNING__QHZ2  QHZ3=tireRL__ALIGNING__QHZ3  QHZ4=tireRL__ALIGNING__QHZ4  PPZ1=tireRL__ALIGNING__PPZ1  PPZ2=tireRL__ALIGNING__PPZ2  SSZ1=tireRL__ALIGNING__SSZ1  SSZ2=tireRL__ALIGNING__SSZ2  SSZ3=tireRL__ALIGNING__SSZ3  SSZ4=tireRL__ALIGNING__SSZ4  PDXP1=tireRL__TURNSLIP__PDXP1  PDXP2=tireRL__TURNSLIP__PDXP2  PDXP3=tireRL__TURNSLIP__PDXP3  PKYP1=tireRL__TURNSLIP__PKYP1  PDYP1=tireRL__TURNSLIP__PDYP1  PDYP2=tireRL__TURNSLIP__PDYP2  PDYP3=tireRL__TURNSLIP__PDYP3  PDYP4=tireRL__TURNSLIP__PDYP4  PHYP1=tireRL__TURNSLIP__PHYP1  PHYP2=tireRL__TURNSLIP__PHYP2  PHYP3=tireRL__TURNSLIP__PHYP3  PHYP4=tireRL__TURNSLIP__PHYP4  PECP1=tireRL__TURNSLIP__PECP1  PECP2=tireRL__TURNSLIP__PECP2  QDTP1=tireRL__TURNSLIP__QDTP1  QCRP1=tireRL__TURNSLIP__QCRP1  QCRP2=tireRL__TURNSLIP__QCRP2  QBRP1=tireRL__TURNSLIP__QBRP1  QDRP1=tireRL__TURNSLIP__QDRP1  QDRP2=tireRL__TURNSLIP__QDRP2  aMode=2
  Combined Slip Wheel 2DOF - RearRight - TUM : vehdynlibtire_TUM/Combined Slip Wheel 2DOF  BrakeType=Disc  mu_static=VEH__Brakes__mue_BrakePadsFrRe_static__2  mu_kinetic=VEH__Brakes__mue_BrakePadsFrRe_kinetic__2  disk_abore=VEH__Brakes__d_BrakeActuatorBoreFrRe_m__2  Rm=VEH__Brakes__r_BrakePadsMeanLeverFrRe_m__2  num_pads=VEH__Brakes__n_BrakePadsNumberFrRe__2  drum_abore=0.0508  drum_a=0.123  drum_c=0.212  drum_r=0.15  drum_theta1=0  drum_theta2=126  brake_p_bpt=[1 11.4736842105263 21.9473684210526 32.4210526315789 42.8947368421053 53.3684210526316 63.8421052631579 74.3157894736842 84.7894736842105 95.2631578947368 105.736842105263 116.210526315789 126.684210526316 137.157894736842 147.631578947368 158.105263157895 168.578947368421 179.052631578947 189.526315789474 200]  brake_n_bpt=[0 52.6315789473684 105.263157894737 157.894736842105 210.526315789474 263.157894736842 315.789473684211 368.421052631579 421.052631578947 473.684210526316 526.315789473684 578.947368421053 631.578947368421 684.210526315789 736.842105263158 789.473684210526 842.105263157895 894.736842105263 947.368421052632 1000]  f_brake_t=[43.4900602404453 42.5056030554862 41.5350898940194 40.5780454442085 39.6340111501808 38.7025443887544 37.7832176914519 36.8756180088306 35.9793460143796 35.0940154454303 34.2192524787115 33.3546951383474 32.4999927342521 31.6548053290159 30.8188032315107 29.991666515561 29.1730845621415 28.362755623661 27.5603864089927 26.765691687993;498.991217495636 487.695866636631 476.560505099801 465.579679307235 454.748127933653 444.060772460445 433.51270824929 423.099196101319 412.81565427025 402.657650900201 392.620896861006 382.701238955775 372.894653477208 363.197240090814 353.605216024701 344.114910546964 334.722759712992 325.425301366216 316.219170376863 307.10109410434;954.492374750826 932.886130217776 911.585920305583 890.581313170261 869.862244717126 849.419000532136 829.242198807128 809.322774193808 789.651962526121 770.221286354971 751.0225412433 732.047782773203 713.289314220164 694.739674852612 676.391628817892 658.238154578366 640.272434863842 622.48784710877 604.877954344734 587.436496520688;1409.99353200602 1378.07639379892 1346.61133551136 1315.58294703329 1284.9763615006 1254.77722860383 1224.97168936497 1195.5463522863 1166.48827078199 1137.78492180974 1109.42418562559 1081.39432659063 1053.68397496312 1026.28210961441 999.178041611083 972.361398609768 945.822110014692 919.550392851325 893.536738312604 867.771898937035;1865.49468926121 1823.26665738007 1781.63675071715 1740.58458089631 1700.09047828407 1660.13545667552 1620.7011799228 1581.76993037878 1543.32457903786 1505.34855726451 1467.82583000789 1430.74087040806 1394.07863570608 1357.82454437621 1321.96445440427 1286.48464264117 1251.37178516554 1216.61293859388 1182.19552228048 1148.10730135338;2320.9958465164 2268.45692096121 2216.66216592293 2165.58621475934 2115.20459506754 2065.49368474721 2016.43067048064 1967.99350847127 1920.16088729373 1872.91219271928 1826.22747439018 1780.08741422549 1734.47329644903 1689.36697913801 1644.75086719747 1600.60788667257 1556.92146031639 1513.67548433643 1470.85430624835 1428.44270376973;2776.49700377159 2713.64718454235 2651.68758112871 2590.58784862237 2530.31871185102 2470.8519128189 2412.16016103848 2354.21708656376 2296.9971955496 2240.47582817405 2184.62911877248 2129.43395804292 2074.86795719199 2020.9094138998 1967.53727999066 1914.73113070398 1862.47113546724 1810.73803007899 1759.51309021622 1708.77810618608;3231.99816102678 3158.8374481235 3086.71299633449 3015.58948248539 2945.43282863449 2876.21014089059 2807.88965159632 2740.44066465625 2673.83350380547 2608.03946362882 2543.03076315477 2478.78050186034 2415.26261793494 2352.4518486616 2290.32369278385 2228.85437473538 2168.02081061809 2107.80057582154 2048.17187418409 1989.11350860242;3687.49931828197 3604.02771170464 3521.73841154027 3440.59111634842 3360.54694541796 3281.56836896228 3203.61914215416 3126.66424274874 3050.66981206134 2975.60309908359 2901.43240753707 2828.12704567777 2755.6572786779 2683.9942834234 2613.11010557704 2542.97761876678 2473.57048576894 2404.8631215641 2336.83065815196 2269.44891101877;4143.00047553716 4049.21797528579 3956.76382674606 3865.59275021144 3775.66106220143 3686.92659703397 3599.34863271199 3512.88782084123 3427.50612031721 3343.16673453836 3259.83405191936 3177.4735894952 3096.05193942085 3015.5367181852 2935.89651837023 2857.10086279818 2779.12016091979 2701.92566730665 2625.48944211983 2549.78431343512;4598.50163279235 4494.40823886693 4391.78924195184 4290.59438407447 4190.77517898491 4092.28482510566 3995.07812326983 3899.11139893372 3804.34242857308 3710.73036999313 3618.23569630166 3526.82013331263 3436.44660016381 3347.079152947 3258.68293116342 3171.22410682959 3084.66983607064 2998.98821304921 2914.1482260877 2830.11971585147;5054.00279004754 4939.59850244808 4826.81465715762 4715.59601793749 4605.88929576838 4497.64305317735 4390.80761382767 4285.3349770262 4181.17873682896 4078.2940054479 3976.63734068395 3876.16667713006 3776.84126090677 3678.62158770879 3581.46934395661 3485.34735086099 ...(+2764 chars)]  tireParamSet=vdynPassCar.mat  plySteer=off  turnslip=off  PRESMAX=tireRR__SIMULATION__PRESMAX  PRESMIN=tireRR__SIMULATION__PRESMIN  FZMAX=tireRR__SIMULATION__FZMAX  FZMIN=tireRR__SIMULATION__FZMIN  VXLOW=tireRR__SIMULATION__VXLOW  KPUMAX=tireRR__SIMULATION__KPUMAX  KPUMIN=tireRR__SIMULATION__KPUMIN  ALPMAX=tireRR__SIMULATION__ALPMAX  ALPMIN=tireRR__SIMULATION__ALPMIN  CAMMAX=tireRR__SIMULATION__CAMMAX  CAMMIN=tireRR__SIMULATION__CAMMIN  LONGVL=tireRR__SIMULATION__LONGVL  omegao=INIT__initialvalues__omega0_Wheels_radps__4  br=tireRR__WHEEL__br_Nmsprad  UNLOADED_RADIUS=tireRR__WHEEL__TYRE_RADIUS_MOD  NOMPRES=tireRR__WHEEL__NORMPRES  FNOMIN=tireRR__WHEEL__FNOMIN  WIDTH=tireRR__DIMENSION__WIDTH  T_RelaxationLong=tireRR__WHEEL__T_RelaxationLong  T_RelaxationLat=tireRR__WHEEL__T_RelaxationLat  T_RelaxationMy=tireRR__WHEEL__T_RelaxationMy  MASS=tireRR__INERTIAL__m_Wheel_kg  IYY=tireRR__INERTIAL__Iyy_Wheel_kgm2  GRAVITY=- VEH__Environment__a_Gravity_mps2  zo=INIT__initialvalues__z0_TireDeflection_m__4  zdoto=INIT__initialvalues__v0z_Wheels_mps__4  BREFF=tireRR__VERTICAL__BREFF  DREFF=tireRR__VERTICAL__DREFF  FREFF=tireRR__VERTICAL__FREFF  Q_RE0=tireRR__VERTICAL__Q_RE0  Q_V1=tireRR__VERTICAL__Q_V1  Q_V2=tireRR__VERTICAL__Q_V2  Q_FZ1=tireRR__VERTICAL__Q_FZ1  Q_FZ2=tireRR__VERTICAL__Q_FZ2  Q_FZ3=tireRR__VERTICAL__Q_FZ3  Q_FCX=tireRR__VERTICAL__Q_FCX  Q_FCY=tireRR__VERTICAL__Q_FCY  Q_FCY2=tireRR__VERTICAL__Q_FCY2  PFZ1=tireRR__VERTICAL__PFZ1  VERTICAL_STIFFNESS=tireRR__VERTICAL__VERTICAL_STIFFNESS  VERTICAL_DAMPING=tireRR__VERTICAL__VERTICAL_DAMPING  LONGITUDINAL_STIFFNESS=tireRR__STRUCTURAL__LONGITUDINAL_STIFFNESS  LATERAL_STIFFNESS=tireRR__STRUCTURAL__LATERAL_STIFFNESS  PCFX1=tireRR__STRUCTURAL__PCFX1  PCFX2=tireRR__STRUCTURAL__PCFX2  PCFX3=tireRR__STRUCTURAL__PCFX3  PCFY1=tireRR__STRUCTURAL__PCFY1  PCFY2=tireRR__STRUCTURAL__PCFY2  PCFY3=tireRR__STRUCTURAL__PCFY3  Q_RA1=tireRR__CONTACTPATCH__Q_RA1  Q_RA2=tireRR__CONTACTPATCH__Q_RA2  Q_RB1=tireRR__CONTACTPATCH__Q_RB1  Q_RB2=tireRR__CONTACTPATCH__Q_RB2  PCX1=tireRR__LONGITUDINAL__PCX1  PDX1=tireRR__LONGITUDINAL__PDX1  PDX2=tireRR__LONGITUDINAL__PDX2  PDX3=tireRR__LONGITUDINAL__PDX3  PEX1=tireRR__LONGITUDINAL__PEX1  PEX2=tireRR__LONGITUDINAL__PEX2  PEX3=tireRR__LONGITUDINAL__PEX3  PEX4=tireRR__LONGITUDINAL__PEX4  PKX1=tireRR__LONGITUDINAL__PKX1  PKX2=tireRR__LONGITUDINAL__PKX2  PKX3=tireRR__LONGITUDINAL__PKX3  PHX1=tireRR__LONGITUDINAL__PHX1  PHX2=tireRR__LONGITUDINAL__PHX2  PVX1=tireRR__LONGITUDINAL__PVX1  PVX2=tireRR__LONGITUDINAL__PVX2  PPX1=tireRR__LONGITUDINAL__PPX1  PPX2=tireRR__LONGITUDINAL__PPX2  PPX3=tireRR__LONGITUDINAL__PPX3  PPX4=tireRR__LONGITUDINAL__PPX4  RBX1=tireRR__LONGITUDINAL__RBX1  RBX2=tireRR__LONGITUDINAL__RBX2  RBX3=tireRR__LONGITUDINAL__RBX3  RCX1=tireRR__LONGITUDINAL__RCX1  REX1=tireRR__LONGITUDINAL__REX1  REX2=tireRR__LONGITUDINAL__REX2  RHX1=tireRR__LONGITUDINAL__RHX1  QSX1=tireRR__OVERTURNING__QSX1  QSX2=tireRR__OVERTURNING__QSX2  QSX3=tireRR__OVERTURNING__QSX3  QSX4=tireRR__OVERTURNING__QSX4  QSX5=tireRR__OVERTURNING__QSX5  QSX6=tireRR__OVERTURNING__QSX6  QSX7=tireRR__OVERTURNING__QSX7  QSX8=tireRR__OVERTURNING__QSX8  QSX9=tireRR__OVERTURNING__QSX9  QSX10=tireRR__OVERTURNING__QSX10  QSX11=tireRR__OVERTURNING__QSX11  QSX12=tireRR__OVERTURNING__QSX12  QSX13=tireRR__OVERTURNING__QSX13  QSX14=tireRR__OVERTURNING__QSX14  PPMX1=tireRR__OVERTURNING__PPMX1  PCY1=tireRR__LATERAL__PCY1  PDY1=tireRR__LATERAL__PDY1  PDY2=tireRR__LATERAL__PDY2  PDY3=tireRR__LATERAL__PDY3  PEY1=tireRR__LATERAL__PEY1  PEY2=tireRR__LATERAL__PEY2  PEY3=tireRR__LATERAL__PEY3  PEY4=tireRR__LATERAL__PEY4  PEY5=tireRR__LATERAL__PEY5  PKY1=tireRR__LATERAL__PKY1  PKY2=tireRR__LATERAL__PKY2  PKY3=tireRR__LATERAL__PKY3  PKY4=tireRR__LATERAL__PKY4  PKY5=tireRR__LATERAL__PKY5  PKY6=tireRR__LATERAL__PKY6  PKY7=tireRR__LATERAL__PKY7  PHY1=tireRR__LATERAL__PHY1  PHY2=tireRR__LATERAL__PHY2  PVY1=tireRR__LATERAL__PVY1  PVY2=tireRR__LATERAL__PVY2  PVY3=tireRR__LATERAL__PVY3  PVY4=tireRR__LATERAL__PVY4  PPY1=tireRR__LATERAL__PPY1  PPY2=tireRR__LATERAL__PPY2  PPY3=tireRR__LATERAL__PPY3  PPY4=tireRR__LATERAL__PPY4  PPY5=tireRR__LATERAL__PPY5  RBY1=tireRR__LATERAL__RBY1  RBY2=tireRR__LATERAL__RBY2  RBY3=tireRR__LATERAL__RBY3  RBY4=tireRR__LATERAL__RBY4  RCY1=tireRR__LATERAL__RCY1  REY1=tireRR__LATERAL__REY1  REY2=tireRR__LATERAL__REY2  RHY1=tireRR__LATERAL__RHY1  RHY2=tireRR__LATERAL__RHY2  RVY1=tireRR__LATERAL__RVY1  RVY2=tireRR__LATERAL__RVY2  RVY3=tireRR__LATERAL__RVY3  RVY4=tireRR__LATERAL__RVY4  RVY5=tireRR__LATERAL__RVY5  RVY6=tireRR__LATERAL__RVY6  QSY1=tireRR__ROLLING__QSY1  QSY2=tireRR__ROLLING__QSY2  QSY3=tireRR__ROLLING__QSY3  QSY4=tireRR__ROLLING__QSY4  QSY5=tireRR__ROLLING__QSY5  QSY6=tireRR__ROLLING__QSY6  QSY7=tireRR__ROLLING__QSY7  QSY8=tireRR__ROLLING__QSY8  QBZ1=tireRR__ALIGNING__QBZ1  QBZ2=tireRR__ALIGNING__QBZ2  QBZ3=tireRR__ALIGNING__QBZ3  QBZ4=tireRR__ALIGNING__QBZ4  QBZ5=tireRR__ALIGNING__QBZ5  QBZ6=tireRR__ALIGNING__QBZ6  QBZ9=tireRR__ALIGNING__QBZ9  QBZ10=tireRR__ALIGNING__QBZ10  QCZ1=tireRR__ALIGNING__QCZ1  QDZ1=tireRR__ALIGNING__QDZ1  QDZ2=tireRR__ALIGNING__QDZ2  QDZ3=tireRR__ALIGNING__QDZ3  QDZ4=tireRR__ALIGNING__QDZ4  QDZ6=tireRR__ALIGNING__QDZ6  QDZ7=tireRR__ALIGNING__QDZ7  QDZ8=tireRR__ALIGNING__QDZ8  QDZ9=tireRR__ALIGNING__QDZ9  QDZ10=tireRR__ALIGNING__QDZ10  QDZ11=tireRR__ALIGNING__QDZ11  QEZ1=tireRR__ALIGNING__QEZ1  QEZ2=tireRR__ALIGNING__QEZ2  QEZ3=tireRR__ALIGNING__QEZ3  QEZ4=tireRR__ALIGNING__QEZ4  QEZ5=tireRR__ALIGNING__QEZ5  QHZ1=tireRR__ALIGNING__QHZ1  QHZ2=tireRR__ALIGNING__QHZ2  QHZ3=tireRR__ALIGNING__QHZ3  QHZ4=tireRR__ALIGNING__QHZ4  PPZ1=tireRR__ALIGNING__PPZ1  PPZ2=tireRR__ALIGNING__PPZ2  SSZ1=tireRR__ALIGNING__SSZ1  SSZ2=tireRR__ALIGNING__SSZ2  SSZ3=tireRR__ALIGNING__SSZ3  SSZ4=tireRR__ALIGNING__SSZ4  PDXP1=tireRR__TURNSLIP__PDXP1  PDXP2=tireRR__TURNSLIP__PDXP2  PDXP3=tireRR__TURNSLIP__PDXP3  PKYP1=tireRR__TURNSLIP__PKYP1  PDYP1=tireRR__TURNSLIP__PDYP1  PDYP2=tireRR__TURNSLIP__PDYP2  PDYP3=tireRR__TURNSLIP__PDYP3  PDYP4=tireRR__TURNSLIP__PDYP4  PHYP1=tireRR__TURNSLIP__PHYP1  PHYP2=tireRR__TURNSLIP__PHYP2  PHYP3=tireRR__TURNSLIP__PHYP3  PHYP4=tireRR__TURNSLIP__PHYP4  PECP1=tireRR__TURNSLIP__PECP1  PECP2=tireRR__TURNSLIP__PECP2  QDTP1=tireRR__TURNSLIP__QDTP1  QCRP1=tireRR__TURNSLIP__QCRP1  QCRP2=tireRR__TURNSLIP__QCRP2  QBRP1=tireRR__TURNSLIP__QBRP1  QDRP1=tireRR__TURNSLIP__QDRP1  QDRP2=tireRR__TURNSLIP__QDRP2  aMode=2
  Manual Switch{,1..3} (4 alike) : ManualSwitch
  Rearrange Signals : Subsystem
  Selector{40..48} (9 alike) : Selector  InputPortWidth=4  IndexOptions=Index vector (dialog)  Indices=1  OutputSizes=1
  Selector49 : Selector  NumberOfDimensions=2  InputPortWidth=4  IndexOptions=Select all,Index vector (dialog)  Indices=1,1  OutputSizes=1,1
  Selector{50..58} (9 alike) : Selector  InputPortWidth=4  IndexOptions=Index vector (dialog)  Indices=2  OutputSizes=1
  Selector59 : Selector  NumberOfDimensions=2  InputPortWidth=4  IndexOptions=Select all,Index vector (dialog)  Indices=2,2  OutputSizes=1,1
  Selector{60..68} (9 alike) : Selector  InputPortWidth=4  IndexOptions=Index vector (dialog)  Indices=3  OutputSizes=1
  Selector69 : Selector  NumberOfDimensions=2  InputPortWidth=4  IndexOptions=Select all,Index vector (dialog)  Indices=3,3  OutputSizes=1,1
  Selector{70..78} (9 alike) : Selector  InputPortWidth=4  IndexOptions=Index vector (dialog)  Indices=4  OutputSizes=1
  Selector79 : Selector  NumberOfDimensions=2  InputPortWidth=4  IndexOptions=Select all,Index vector (dialog)  Indices=4,4  OutputSizes=1,1
  Terminator{21,29..55} (28 alike) : Terminator
  Fx [1x4] : Outport
  Fy [1x4] : Outport  Port=2
  Fz [1x4] : Outport  Port=3
  Mx [1x4] : Outport  Port=4
  My [1x4] : Outport  Port=5
  Mz [1x4] : Outport  Port=6
  z [1x4] : Outport  Port=7
  zdot [1x4] : Outport  Port=8
  Re [1x4] : Outport  Port=9
  omega [1x4] : Outport  Port=10
  Kappa [1x4] : Outport  Port=11
  Alpha [1x4] : Outport  Port=12
  wires:
  BrkPrs [1x4]/1 -> Bus Creator/1  "BrkPrs"
  AxlTrq [1x4]/1 -> Bus Creator/2  "AxlTrq"
  Vx [1x4]/1 -> Bus Creator/3  "Vx"
  Vy [1x4]/1 -> Bus Creator/4  "Vy"
  Camber [1x4]/1 -> Bus Creator/5  "Camber"
  YawRate [1x4]/1 -> Bus Creator/6  "YawRate"
  Prs [1x4]/1 -> Bus Creator/7  "Prs"
  Gnd [1x4]/1 -> Bus Creator/8  "Gnd"
  Fext [1x4]/1 -> Bus Creator/9  "Fext"
  ScaleFctrs [27x4]/1 -> Bus Creator/10  "ScaleFctrs"
  Rearrange Signals/8(z) -> z [1x4]/1
  Rearrange Signals/10(Re) -> Re [1x4]/1
  Rearrange Signals/5(Mx) -> Mx [1x4]/1
  Rearrange Signals/4(Fz) -> Fz [1x4]/1
  Rearrange Signals/3(Fy) -> Fy [1x4]/1
  Rearrange Signals/7(Mz) -> Mz [1x4]/1
  Rearrange Signals/6(My) -> My [1x4]/1
  Rearrange Signals/9(zdot) -> zdot [1x4]/1
  Rearrange Signals/2(Fx) -> Fx [1x4]/1
  Rearrange Signals/1(omega) -> omega [1x4]/1
  Rearrange Signals/11(Kappa) -> Kappa [1x4]/1
  Rearrange Signals/12(Alpha) -> Alpha [1x4]/1
  Selector49/1 -> Combined Slip Wheel 2DOF - FrontLeft - TUM1/10
  Selector48/1 -> Combined Slip Wheel 2DOF - FrontLeft - TUM1/9
  Selector47/1 -> Combined Slip Wheel 2DOF - FrontLeft - TUM1/8
  Selector45/1 -> Combined Slip Wheel 2DOF - FrontLeft - TUM1/6
  Selector42/1 -> Combined Slip Wheel 2DOF - FrontLeft - TUM1/3
  Bus Selector4/7 -> Selector46/1  "<Prs>"
  Bus Selector4/3 -> Selector42/1  "<Vx>"
  Bus Selector4/8 -> Selector47/1  "<Gnd>"
  Bus Selector4/10 -> Selector49/1  "<ScaleFctrs>"
  Bus Selector4/9 -> Selector48/1  "<Fext>"
  Bus Selector4/5 -> Selector44/1  "<Camber>"
  Bus Selector4/1 -> Selector40/1  "<BrkPrs>"
  Bus Selector4/2 -> Selector41/1  "<AxlTrq>"
  Selector41/1 -> Combined Slip Wheel 2DOF - FrontLeft - TUM1/2
  Selector44/1 -> Combined Slip Wheel 2DOF - FrontLeft - TUM1/5
  Bus Selector4/4 -> Selector43/1  "<Vy>"
  Selector46/1 -> Combined Slip Wheel 2DOF - FrontLeft - TUM1/7
  Selector40/1 -> Combined Slip Wheel 2DOF - FrontLeft - TUM1/1
  Bus Selector4/6 -> Selector45/1  "<YawRate>"
  Selector43/1 -> Combined Slip Wheel 2DOF - FrontLeft - TUM1/4
  Bus Selector5/7 -> Selector56/1  "<Prs>"
  Bus Selector5/10 -> Selector59/1  "<ScaleFctrs>"
  Bus Selector5/1 -> Selector50/1  "<BrkPrs>"
  Bus Selector5/9 -> Selector58/1  "<Fext>"
  Bus Selector5/3 -> Selector52/1  "<Vx>"
  Bus Selector5/6 -> Selector55/1  "<YawRate>"
  Bus Selector5/4 -> Selector53/1  "<Vy>"
  Bus Selector5/5 -> Selector54/1  "<Camber>"
  Bus Selector5/8 -> Selector57/1  "<Gnd>"
  Selector54/1 -> Combined Slip Wheel 2DOF - FrontRight - TUM1/5
  Selector59/1 -> Combined Slip Wheel 2DOF - FrontRight - TUM1/10
  Bus Selector5/2 -> Selector51/1  "<AxlTrq>"
  Selector52/1 -> Combined Slip Wheel 2DOF - FrontRight - TUM1/3
  Selector55/1 -> Combined Slip Wheel 2DOF - FrontRight - TUM1/6
  Selector50/1 -> Combined Slip Wheel 2DOF - FrontRight - TUM1/1
  Selector57/1 -> Combined Slip Wheel 2DOF - FrontRight - TUM1/8
  Selector51/1 -> Combined Slip Wheel 2DOF - FrontRight - TUM1/2
  Selector53/1 -> Combined Slip Wheel 2DOF - FrontRight - TUM1/4
  Selector56/1 -> Combined Slip Wheel 2DOF - FrontRight - TUM1/7
  Selector58/1 -> Combined Slip Wheel 2DOF - FrontRight - TUM1/9
  Selector61/1 -> Combined Slip Wheel 2DOF - RearLeft - TUM/2
  Bus Selector6/4 -> Selector63/1  "<Vy>"
  Bus Selector6/3 -> Selector62/1  "<Vx>"
  Bus Selector6/10 -> Selector69/1  "<ScaleFctrs>"
  Bus Selector6/1 -> Selector60/1  "<BrkPrs>"
  Bus Selector6/2 -> Selector61/1  "<AxlTrq>"
  Bus Selector6/7 -> Selector66/1  "<Prs>"
  Selector65/1 -> Combined Slip Wheel 2DOF - RearLeft - TUM/6
  Selector64/1 -> Combined Slip Wheel 2DOF - RearLeft - TUM/5
  Selector68/1 -> Combined Slip Wheel 2DOF - RearLeft - TUM/9
  Bus Selector6/5 -> Selector64/1  "<Camber>"
  Bus Selector6/6 -> Selector65/1  "<YawRate>"
  Selector67/1 -> Combined Slip Wheel 2DOF - RearLeft - TUM/8
  Selector69/1 -> Combined Slip Wheel 2DOF - RearLeft - TUM/10
  Selector60/1 -> Combined Slip Wheel 2DOF - RearLeft - TUM/1
  Bus Selector6/9 -> Selector68/1  "<Fext>"
  Bus Selector6/8 -> Selector67/1  "<Gnd>"
  Selector63/1 -> Combined Slip Wheel 2DOF - RearLeft - TUM/4
  Bus Creator/1 -> Bus Selector7/1, Bus Selector5/1, Bus Selector6/1, Bus Selector4/1
  Selector62/1 -> Combined Slip Wheel 2DOF - RearLeft - TUM/3
  Selector66/1 -> Combined Slip Wheel 2DOF - RearLeft - TUM/7
  Bus Selector7/8 -> Selector77/1  "<Gnd>"
  Bus Selector7/1 -> Selector70/1  "<BrkPrs>"
  Bus Selector7/3 -> Selector72/1  "<Vx>"
  Bus Selector7/6 -> Selector75/1  "<YawRate>"
  Bus Selector7/4 -> Selector73/1  "<Vy>"
  Bus Selector7/2 -> Selector71/1  "<AxlTrq>"
  Bus Selector7/10 -> Selector79/1  "<ScaleFctrs>"
  Bus Selector7/7 -> Selector76/1  "<Prs>"
  Selector79/1 -> Combined Slip Wheel 2DOF - RearRight - TUM/10
  Selector77/1 -> Combined Slip Wheel 2DOF - RearRight - TUM/8
  Selector78/1 -> Combined Slip Wheel 2DOF - RearRight - TUM/9
  Selector74/1 -> Combined Slip Wheel 2DOF - RearRight - TUM/5
  Bus Selector7/9 -> Selector78/1  "<Fext>"
  Selector75/1 -> Combined Slip Wheel 2DOF - RearRight - TUM/6
  Selector72/1 -> Combined Slip Wheel 2DOF - RearRight - TUM/3
  Selector76/1 -> Combined Slip Wheel 2DOF - RearRight - TUM/7
  Selector73/1 -> Combined Slip Wheel 2DOF - RearRight - TUM/4
  Selector71/1 -> Combined Slip Wheel 2DOF - RearRight - TUM/2
  Bus Selector7/5 -> Selector74/1  "<Camber>"
  Selector70/1 -> Combined Slip Wheel 2DOF - RearRight - TUM/1
  Combined Slip Wheel 2DOF - RearLeft - TUM/6 -> Terminator32/1
  Combined Slip Wheel 2DOF - RearLeft - TUM/3 -> Terminator29/1
  Combined Slip Wheel 2DOF - RearLeft - TUM/2 -> Terminator21/1
  Combined Slip Wheel 2DOF - RearLeft - TUM/5 -> Terminator31/1
  Combined Slip Wheel 2DOF - RearLeft - TUM/4 -> Terminator30/1
  Combined Slip Wheel 2DOF - RearLeft - TUM/7 -> Terminator33/1
  Combined Slip Wheel 2DOF - RearLeft - TUM/8 -> Terminator34/1
  Combined Slip Wheel 2DOF - RearRight - TUM/6 -> Terminator39/1
  Combined Slip Wheel 2DOF - RearRight - TUM/3 -> Terminator36/1
  Combined Slip Wheel 2DOF - RearRight - TUM/2 -> Terminator35/1
  Combined Slip Wheel 2DOF - RearRight - TUM/5 -> Terminator38/1
  Combined Slip Wheel 2DOF - RearRight - TUM/4 -> Terminator37/1
  Combined Slip Wheel 2DOF - RearRight - TUM/7 -> Terminator40/1
  Combined Slip Wheel 2DOF - RearRight - TUM/8 -> Terminator41/1
  Combined Slip Wheel 2DOF - FrontRight - TUM1/6 -> Terminator46/1
  Combined Slip Wheel 2DOF - FrontRight - TUM1/3 -> Terminator43/1
  Combined Slip Wheel 2DOF - FrontRight - TUM1/2 -> Terminator42/1
  Combined Slip Wheel 2DOF - FrontRight - TUM1/5 -> Terminator45/1
  Combined Slip Wheel 2DOF - FrontRight - TUM1/4 -> Terminator44/1
  Combined Slip Wheel 2DOF - FrontRight - TUM1/7 -> Terminator47/1
  Combined Slip Wheel 2DOF - FrontRight - TUM1/8 -> Terminator48/1
  Combined Slip Wheel 2DOF - FrontLeft - TUM1/6 -> Terminator53/1
  Combined Slip Wheel 2DOF - FrontLeft - TUM1/3 -> Terminator50/1
  Combined Slip Wheel 2DOF - FrontLeft - TUM1/2 -> Terminator49/1
  Combined Slip Wheel 2DOF - FrontLeft - TUM1/5 -> Terminator52/1
  Combined Slip Wheel 2DOF - FrontLeft - TUM1/4 -> Terminator51/1
  Combined Slip Wheel 2DOF - FrontLeft - TUM1/7 -> Terminator54/1
  Combined Slip Wheel 2DOF - FrontLeft - TUM1/8 -> Terminator55/1
  Combined Slip Wheel 2DOF - RearLeft - TUM/1 -> Manual Switch2/1
  Combined Slip Wheel 2DOF - FrontLeft - TUM1/1 -> Manual Switch/1
  Combined Slip Wheel 2DOF - FrontRight - TUM1/1 -> Manual Switch3/1
  Combined Slip Wheel 2DOF - RearRight - TUM/1 -> Manual Switch1/1
  Manual Switch1/1 -> Rearrange Signals/4(Info_rr)
  Manual Switch2/1 -> Rearrange Signals/3(Info_rl)
  Manual Switch3/1 -> Rearrange Signals/2(Info_fr)
  Manual Switch/1 -> Rearrange Signals/1(Info_fl)
